simulink model "gm_CALC_MODEL_FLOAT"  (R2022a)
settings: Solver=VariableStepAuto  StartTime=0.0  StopTime=10.0  RelTol=1e-3
settings Model: Creator=Mykyta  LastModifiedBy=Mykyta
settings OptimizationCC: BlockReduction=off  ConditionallyExecuteInputs=off
settings DebuggingCC: InheritedTsInSrcMsg=none

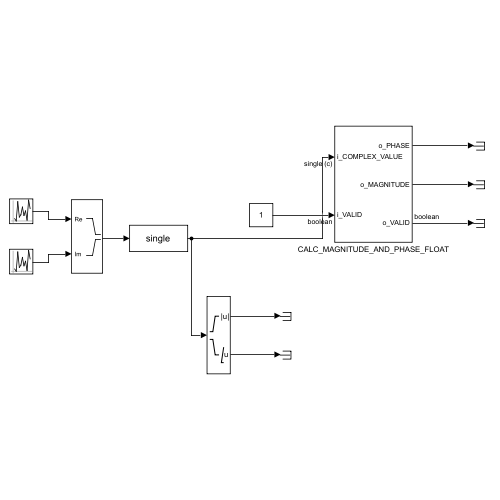
[thumbnail: Simulink's stored preview of the top-level diagram]
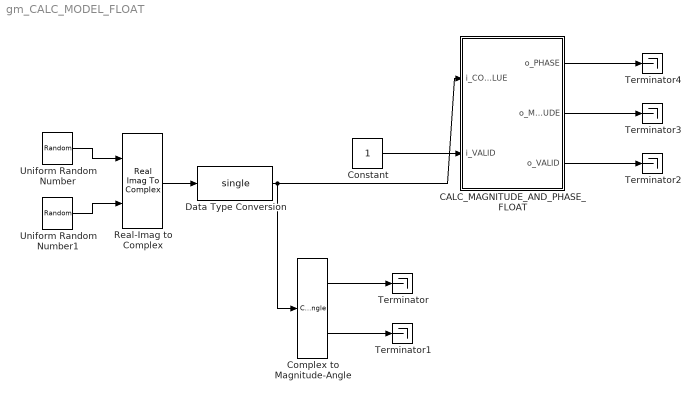
== system gm_CALC_MODEL_FLOAT ==
  CALC_MAGNITUDE_AND_PHASE_FLOAT : Subsystem
  Complex to Magnitude-Angle : ComplexToMagnitudeAngle
  Constant : Constant  OutDataTypeStr=boolean  SampleTime=1
  Data Type Conversion : DataTypeConversion  OutDataTypeStr=single  SaturateOnIntegerOverflow=off  RndMeth=Floor
  Real-Imag to Complex : RealImagToComplex
  Terminator{,1..4} (5 alike) : Terminator
  Uniform Random Number : UniformRandomNumber  Minimum=0  Maximum=16383.999996185302734375  Seed=14  SampleTime=1
  Uniform Random Number1 : UniformRandomNumber  Minimum=0  Maximum=16383.999996185302734375  Seed=15  SampleTime=1
  wires:
  Data Type Conversion/1 -> Complex to Magnitude-Angle/1, CALC_MAGNITUDE_AND_PHASE_FLOAT/1(i_COMPLEX_VALUE)
  Real-Imag to Complex/1 -> Data Type Conversion/1
  CALC_MAGNITUDE_AND_PHASE_FLOAT/3(o_VALID) -> Terminator2/1
  Constant/1 -> CALC_MAGNITUDE_AND_PHASE_FLOAT/2(i_VALID)
  CALC_MAGNITUDE_AND_PHASE_FLOAT/2(o_MAGNITUDE) -> Terminator3/1
  CALC_MAGNITUDE_AND_PHASE_FLOAT/1(o_PHASE) -> Terminator4/1
  Complex to Magnitude-Angle/1 -> Terminator/1
  Complex to Magnitude-Angle/2 -> Terminator1/1
  Uniform Random Number1/1 -> Real-Imag to Complex/2
  Uniform Random Number/1 -> Real-Imag to Complex/1

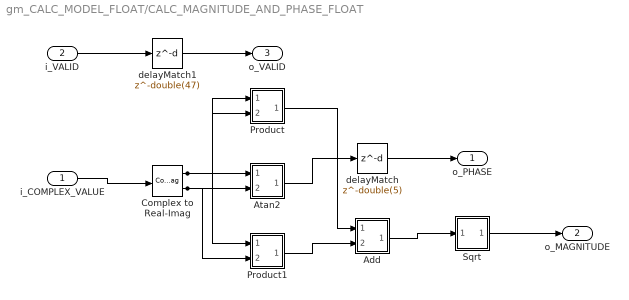
== system gm_CALC_MODEL_FLOAT/CALC_MAGNITUDE_AND_PHASE_FLOAT ==
  i_COMPLEX_VALUE : Inport  OutDataTypeStr=single  PortDimensions=1  SampleTime=1
      settings: SignalType=complex
  i_VALID : Inport  Port=2  OutDataTypeStr=boolean  PortDimensions=1  SampleTime=1
  Add : Subsystem
      mask Display: disp('NFP\nadd');
  Atan2 : Subsystem
      mask Display: disp('NFP\ntrig3');
  Complex to Real-Imag : ComplexToRealImag  SampleTime=1
  Product : Subsystem
      mask Display: disp('NFP\nmul');
  Product1 : Subsystem
      mask Display: disp('NFP\nmul');
  Sqrt : Subsystem
      mask Display: disp('NFP\nsqrt');
  delayMatch : Delay  DelayLength=double(5)  InitialCondition=0  SampleTime=1
  delayMatch1 : Delay  DelayLength=double(47)  InitialCondition=0  SampleTime=1
  o_PHASE : Outport  SampleTime=1
  o_MAGNITUDE : Outport  Port=2  SampleTime=1
  o_VALID : Outport  Port=3  OutDataTypeStr=boolean  SampleTime=1
  wires:
  i_COMPLEX_VALUE/1 -> Complex to Real-Imag/1
  delayMatch1/1 -> o_VALID/1
  delayMatch/1 -> o_PHASE/1
  Complex to Real-Imag/1 -> Product/2(In2), Product/1(In1), Atan2/2(In2)
  Complex to Real-Imag/2 -> Product1/2(In2), Product1/1(In1), Atan2/1(In1)
  Add/1(Out1) -> Sqrt/1(In1)
  Atan2/1(Out1) -> delayMatch/1
  Product/1(Out1) -> Add/1(In1)
  Product1/1(Out1) -> Add/2(In2)
  Sqrt/1(Out1) -> o_MAGNITUDE/1
  i_VALID/1 -> delayMatch1/1

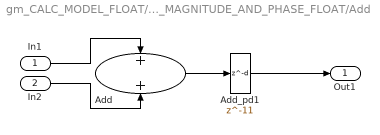
== system gm_CALC_MODEL_FLOAT/CALC_MAGNITUDE_AND_PHASE_FLOAT/Add ==
  In1 : Inport
  In2 : Inport  Port=2
  Add : Sum  OutDataTypeStr=single  SampleTime=1
  Add_pd1 : Delay  DelayLength=11
  Out1 : Outport
  wires:
  In1/1 -> Add/1
  In2/1 -> Add/2
  Add/1 -> Add_pd1/1
  Add_pd1/1 -> Out1/1

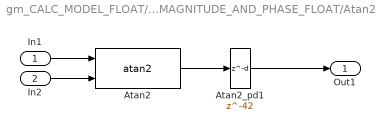
== system gm_CALC_MODEL_FLOAT/CALC_MAGNITUDE_AND_PHASE_FLOAT/Atan2 ==
  In1 : Inport
  In2 : Inport  Port=2
  Atan2 : Trigonometry  Operator=atan2  SampleTime=1
  Atan2_pd1 : Delay  DelayLength=42
  Out1 : Outport
  wires:
  In1/1 -> Atan2/1
  In2/1 -> Atan2/2
  Atan2/1 -> Atan2_pd1/1
  Atan2_pd1/1 -> Out1/1

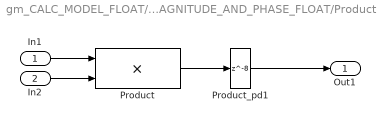
== system gm_CALC_MODEL_FLOAT/CALC_MAGNITUDE_AND_PHASE_FLOAT/Product ==
  In1 : Inport
  In2 : Inport  Port=2
  Product : Product  Inputs=**  OutDataTypeStr=single  SaturateOnIntegerOverflow=on  SampleTime=1
  Product_pd1 : Delay  DelayLength=8
  Out1 : Outport
  wires:
  In1/1 -> Product/1
  In2/1 -> Product/2
  Product/1 -> Product_pd1/1
  Product_pd1/1 -> Out1/1

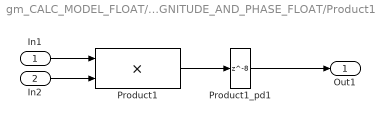
== system gm_CALC_MODEL_FLOAT/CALC_MAGNITUDE_AND_PHASE_FLOAT/Product1 ==
  In1 : Inport
  In2 : Inport  Port=2
  Product1 : Product  Inputs=**  OutDataTypeStr=single  SampleTime=1
  Product1_pd1 : Delay  DelayLength=8
  Out1 : Outport
  wires:
  In1/1 -> Product1/1
  In2/1 -> Product1/2
  Product1/1 -> Product1_pd1/1
  Product1_pd1/1 -> Out1/1

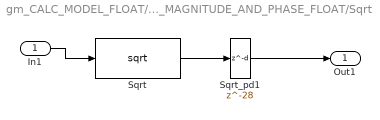
== system gm_CALC_MODEL_FLOAT/CALC_MAGNITUDE_AND_PHASE_FLOAT/Sqrt ==
  In1 : Inport
  Sqrt : Sqrt  SampleTime=1
  Sqrt_pd1 : Delay  DelayLength=28
  Out1 : Outport
  wires:
  In1/1 -> Sqrt/1
  Sqrt/1 -> Sqrt_pd1/1
  Sqrt_pd1/1 -> Out1/1
